simulink model "PIDZieglerNichols"  (R2014a)
settings: Solver=ode45  StartTime=0.0  StopTime=500  RelTol=1e-3
settings Model: Creator=tri  LastModifiedBy=tri

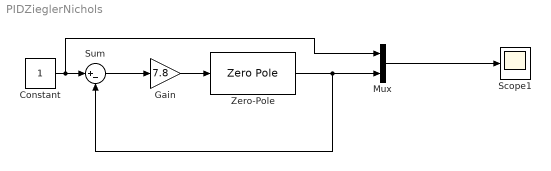
== system PIDZieglerNichols ==
  Constant : Constant
  Gain : Gain  Gain=7.8
  Mux : Mux  Inputs=2
  Scope1 : Scope
  Sum : Sum  Inputs=|+-
  Zero-Pole : ZeroPole  Zeros=[]  Poles=[-1 -0.1 -0.2 ]  Gain=0.05
  wires:
  Gain/1 -> Zero-Pole/1
  Zero-Pole/1 -> Mux/2, Sum/2
  Mux/1 -> Scope1/1
  Constant/1 -> Mux/1, Sum/1
  Sum/1 -> Gain/1
